simulink model "twolink_frty"  (R2017b)
settings: Solver=VariableStepAuto  StartTime=0.0  StopTime=20  RelTol=1e-3
libraries: roblocks x2
settings Model: Creator=sathish  LastModifiedBy=sathish

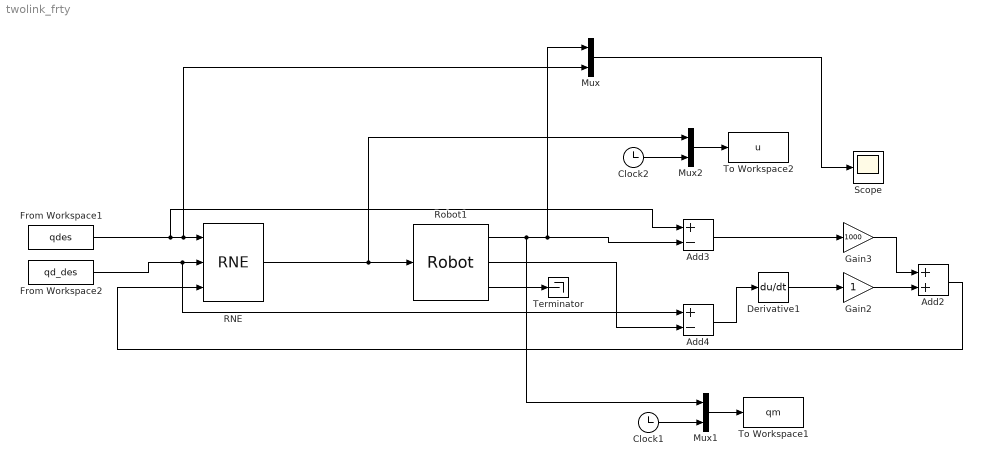
== system twolink_frty ==
  Add2 : Sum
  Add3 : Sum  Inputs=+-
  Add4 : Sum  Inputs=+-
  Clock1 : Clock
  Clock2 : Clock
  Derivative1 : Derivative
  From Workspace1 : FromWorkspace  VariableName=qdes  SampleTime=0.05
  From Workspace2 : FromWorkspace  VariableName=qd_des  SampleTime=0.05
  Gain2 : Gain
  Gain3 : Gain  Gain=1000
  Mux : Mux  Inputs=2
  Mux1 : Mux  Inputs=2
  Mux2 : Mux  Inputs=2
  RNE : roblocks/Arm/RNE  robot=twolink_n  grav=[0 0 -9.81]
  Robot1 : roblocks/Arm/Robot  robot=twolink  q0=[0 0]
  Scope : Scope
  Terminator : Terminator
  To Workspace1 : ToWorkspace  VariableName=qm  SaveFormat=Timeseries  SampleTime=0.05
  To Workspace2 : ToWorkspace  VariableName=u  SaveFormat=Timeseries  SampleTime=0.05
  wires:
  From Workspace2/1 -> Add4/1, RNE/2
  Gain2/1 -> Add2/2
  Derivative1/1 -> Gain2/1
  From Workspace1/1 -> Add3/1, Mux/2, RNE/1
  Gain3/1 -> Add2/1
  Add3/1 -> Gain3/1
  Robot1/2 -> Add4/2
  Add4/1 -> Derivative1/1
  Add2/1 -> RNE/3
  Mux1/1 -> To Workspace1/1
  Clock1/1 -> Mux1/2
  Mux2/1 -> To Workspace2/1
  Clock2/1 -> Mux2/2
  RNE/1 -> Mux2/1, Robot1/1
  Robot1/3 -> Terminator/1
  Robot1/1 -> Mux1/1, Mux/1, Add3/2
  Mux/1 -> Scope/1
